simulink model "motor_simulink_model"  (R2018b)
settings: Solver=VariableStepAuto  StartTime=0.0  StopTime=10.0  RelTol=1e-3
settings Model: Creator=luonc  LastModifiedBy=luonc

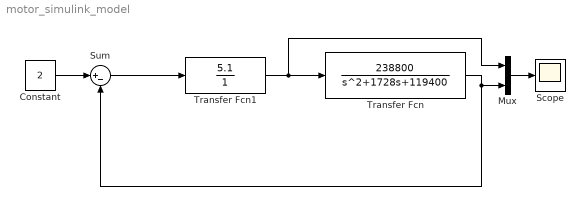
== system motor_simulink_model ==
  Constant : Constant  Value=2  SampleTime=0.5
  Mux : Mux  Inputs=2
  Scope : Scope
  Sum : Sum  Inputs=|+-
  Transfer Fcn : TransferFcn  Numerator=[238800]  Denominator=[1 1728 119400]
  Transfer Fcn1 : TransferFcn  Numerator=[5.1]  Denominator=[1]
  wires:
  Sum/1 -> Transfer Fcn1/1
  Transfer Fcn/1 -> Mux/2, Sum/2
  Constant/1 -> Sum/1
  Transfer Fcn1/1 -> Mux/1, Transfer Fcn/1
  Mux/1 -> Scope/1
